simulink model "PID"  (R2017a)
settings: Solver=ode45  StartTime=0.0  StopTime=10  FixedStep=0.05  MaxStep=0.05  RelTol=1e-3
libraries: simulink x1
settings Model: Creator=asus  LastModifiedBy=Lenovo

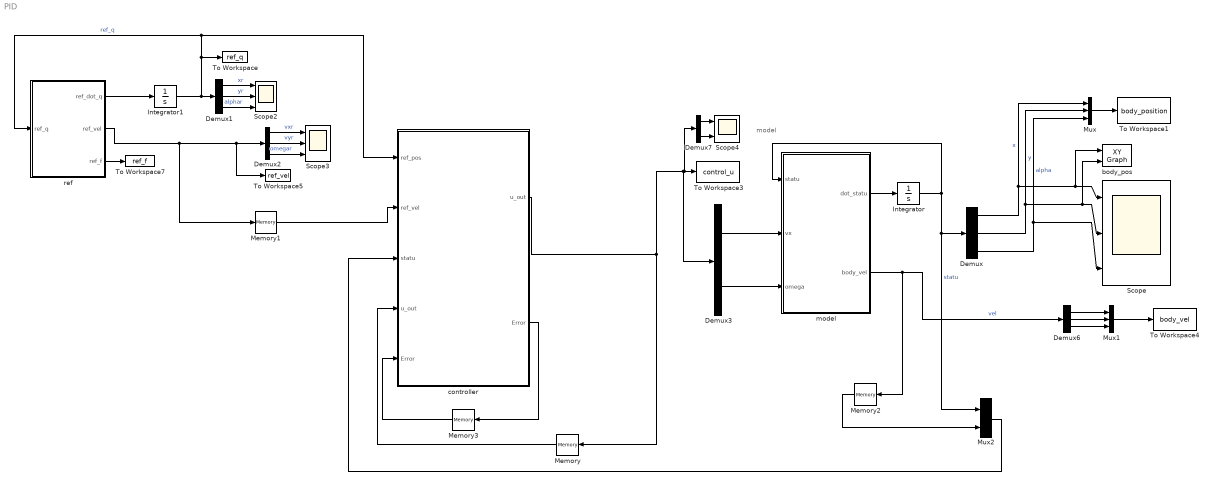
== system PID ==
  note: model
  Demux{,1..2,6} (4 alike) : Demux  Outputs=3
  Demux3 : Demux  Outputs=2
  Demux7 : Demux  Outputs=2
  Integrator : Integrator  InitialCondition=[0; 0; pi/4;]  IgnoreLimit=on
  Integrator1 : Integrator  InitialCondition=[0;0;pi/4]
  Memory : Memory  X0=[0; 0]
  Memory1 : Memory  X0=[0.00001; 0.00001 ; 0.000001]
  Memory2 : Memory  X0=[0.001 0 0]
  Memory3 : Memory  X0=[0 0 0 0]
  Mux : Mux  Inputs=3
  Mux1 : Mux  Inputs=3
  Mux2 : Mux  Inputs=2
  Scope : Scope  NumInputPorts=3
  Scope2 : Scope  NumInputPorts=3
  Scope3 : Scope  NumInputPorts=3
  Scope4 : Scope  NumInputPorts=2
  To Workspace : ToWorkspace  VariableName=ref_q  SampleTime=-1
  To Workspace1 : ToWorkspace  VariableName=body_position  SampleTime=-1
  To Workspace3 : ToWorkspace  VariableName=control_u  SampleTime=-1
  To Workspace4 : ToWorkspace  VariableName=body_vel  SampleTime=-1
  To Workspace5 : ToWorkspace  VariableName=ref_vel  SampleTime=-1
  To Workspace7 : ToWorkspace  VariableName=ref_f  SampleTime=-1
  body_pos : simulink/Sinks/XY Graph  xmin=-10  xmax=10  ymin=-10  ymax=10  st=-1
  controller : MATLAB Function  TreatAsAtomicUnit=on
  model : MATLAB Function  TreatAsAtomicUnit=on
  ref : MATLAB Function  TreatAsAtomicUnit=on
  wires:
  Demux2/2 -> Scope3/2  "vyr"
  Demux2/1 -> Scope3/1  "vxr"
  ref/2(ref_vel) -> Memory1/1, To Workspace5/1, Demux2/1
  Integrator/1 -> Demux/1, Mux2/1, model/1(statu)  "statu"
  Demux1/3 -> Scope2/3  "alphar"
  Demux1/1 -> Scope2/1  "xr"
  Demux1/2 -> Scope2/2  "yr"
  Demux2/3 -> Scope3/3  "omegar"
  Demux/3 -> Mux/3, Scope/3  "alpha"
  Demux/1 -> Mux/1, body_pos/1, Scope/1  "x"
  Demux/2 -> Mux/2, body_pos/2, Scope/2  "y"
  ref/1(ref_dot_q) -> Integrator1/1
  Integrator1/1 -> ref/1(ref_q), controller/1(ref_pos), To Workspace/1, Demux1/1  "ref_q"
  Demux7/2 -> Scope4/2
  Demux7/1 -> Scope4/1
  model/1(dot_statu) -> Integrator/1
  Demux3/1 -> model/2(vx)
  controller/1(u_out) -> Demux7/1, To Workspace3/1, Demux3/1, Memory/1
  Demux3/2 -> model/3(omega)
  Mux1/1 -> To Workspace4/1
  Mux/1 -> To Workspace1/1
  Memory/1 -> controller/4("u_out ")
  Memory1/1 -> controller/2(ref_vel)
  ref/3(ref_f) -> To Workspace7/1
  Demux6/2 -> Mux1/2
  Demux6/1 -> Mux1/1
  Demux6/3 -> Mux1/3
  Mux2/1 -> controller/3(statu)
  Memory2/1 -> Mux2/2
  model/2(body_vel) -> Memory2/1, Demux6/1  "vel"
  controller/2(Error) -> Memory3/1
  Memory3/1 -> controller/5("Error ")

== matlab function PID/controller ==
  data: ref_pos input; ref_vel input; u_out output; statu input; u_out input; Error input; Error output
function [u_out,Error] = my__controller(ref_pos, ref_vel, statu, u_out,Error)
% 程序上没有问题，在运动学模型上是可以完成任务的
% 最近修改时间：11. 20
% 基于运动学模型的   控制器
% u_out=[vx ;  omega]
% ref_vel=[xr yr alphar vr omegar]
% e = [ex ey ealpha]


%% 测试是否能得到
%    statu=[2; -2; pi/2; 0.001; 0.001; 0.001];
%    u_out=[0; 0];
%    ref_pos=[0;0;pi/4]; ref_vel=[2; 0; 0];  
%    Error=[0 0 0 0];
%% 底盘参数
% d = 0.18;	l = 0.16;	m = 24;	Iz = 11.89;	c = 513.6; %轮胎侧偏刚度

%% 状态量                                                                           
x = statu(1);   y = statu(2);  alpha = statu(3); 
vx = statu(4);  vy = statu(5);    omega = statu(6);

xr=ref_pos(1);  yr=ref_pos(2);  alphar=ref_pos(3);
vxr=ref_vel(1); vyr=ref_vel(2); omegar=ref_vel(3);

e1k_1=Error(1);    e1k_2=Error(2);
e2k_1=Error(2);    e2k_2=Error(3);


%%  误差
ex=x-xr;    ey=y-yr;    ealpha=alpha-alphar;
ev=vx-vxr;  eomega=omega-omegar;


 e1k=ex*ex+ey*ey;
 kp1=  0.4  ;   ki1= 0.4   ;   kd1=  0.4  ;
% delta_vx=kp1*(e1k-e1k_1)+ki1*e1k+kd1*(e1k-2*e1k_1+e1k_2);
delta_vx=0.5;

e2k=ealpha*ealpha;
kp2=0.4;  ki2=0.4;  kd2=0.4;
delta_omega=kp2*(e2k-e2k_1)+ki2*e2k+kd2*(e2k-2*e2k_1+e2k_2);

delta_uout=[delta_vx;delta_omega];

u_out = delta_uout+u_out;

e1k_2=e1k_1;
e1k_1=e1k;

e2k_2=e2k_1;
e2k_1=e2k;

Error=[e1k_1;   e1k_2;   e2k_1 ;   e2k_2];

== matlab function PID/model ==
  data: statu input; vx input; dot_statu output; omega input; body_vel output
function [dot_statu, body_vel] = model(statu, vx ,omega)

x = statu(1);
y = statu(2);
alpha = statu(3);

dot_x = vx*cos(alpha);
dot_y = vx*sin(alpha);
dot_alpha = omega;



% 状态【x y alpha vx vy omega】
dot_statu = [dot_x; dot_y; dot_alpha];
vy=0;
body_vel=[vx;vy; omega]


end

% max=1/wheel_radius;
% for i=1:size(wheel_omega,2)
%     if wheel_omega(i)>max
%         wheel_omega(i) = max;
%     else
%         if wheel_omega(i)<-max
%             wheel_omega(i) = -max;
%         else
%             wheel_omega(i) = wheel_omega(i);
%         end
%     end
% end

== matlab function PID/ref ==
  data: ref_q input; ref_dot_q output; ref_vel output; ref_f output
%参考轨迹
%更改时，只需更改vx和Omega即可，实现圆形和直线的不同变化



function [ref_dot_q,ref_vel,ref_f] = fcn(ref_q)
xr=ref_q(1);
yr=ref_q(2);
alphar=ref_q(3);

vxr=1;
vyr=0;
omegar=0.5;

ref_vel=[vxr;vyr;omegar];

dotx = vxr*cos(alphar) - vyr*sin(alphar);
doty = vxr*sin(alphar) + vyr*sin(alphar);
dotalpha = omegar;
ref_dot_q=[dotx;doty;dotalpha];

ref_f = [0;0]
end
